simulink library "AerialManipulation"  (R2016b)
settings: Solver=VariableStepAuto  StartTime=0.0  StopTime=10.0  RelTol=1e-3
undefined symbols (not defined in the file): l
libraries: AerialManipulation x4, aerolibutil x2
settings Model: Creator=Administrator  LastModifiedBy=Administrator

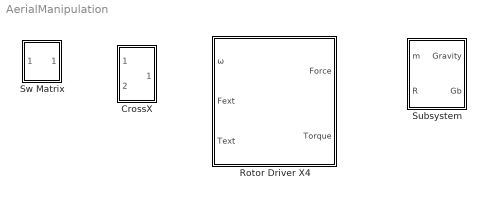
== system AerialManipulation ==
  CrossX : Subsystem
      mask help: 实现向量叉乘 V×P
      mask Display: fprintf('×\nCross');
  Rotor Driver X4 : Subsystem  mask{l=0.18, Fe=[ [0;0;1],[0;0;1],[0;0;1],[0;0;1] ], r=[ [l;0;0],[0;l;0],[-l;0;0],[0;-l;0] ], Td=[ [0;0;1], [0;0;-1],[0;0;1],[0;0;-1] ], Kct=3.16e-05, Ktf=0.01}
      mask prompts: l "length of Arm of force"; Fe "direction of vector"; r "position the force"; Td "direction of counter torque"; Kct "coefficient of counter torque"; Ktf "coefficient of thrust force"
      mask help:
      | 四旋翼的驱动模型
      | 根据四个电机的转速ω计算相应的力与力矩
      mask Display:
      | fprintf('RotorDriverX4');
      | port_label('input',1,'ω','texmode','on');
      | port_label('input',2,'Fext','texmode','on');
      | port_label('input',3,'Text','texmode','on');
      | 
      | port_label('output',1,'F','texmode','on');
      | port_label('output',2,'Torque','texmode','on');
  Subsystem : Subsystem
      mask help: 根据质量m和旋转矩阵R计算重力G和在刚体下的表示Gb
      mask Display:
      | fprintf('Gravity');
      | port_label('input',1,'m','texmode','on');
      | port_label('input',2,'R','texmode','on');
      | 
      | port_label('output',1,'G','texmode','on');
      | port_label('output',2,'Gb','texmode','on');
  Sw Matrix : Subsystem
      mask help:
      | 将一个3×1 v 的向量转为3×3矩阵Sw(v)
      | v×P=Sw(v)P
      | 参看《机器人学导论》P111 (5-25)式子
      mask Display: fprintf('Sw');

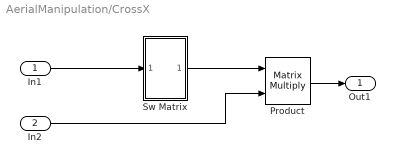
== system AerialManipulation/CrossX ==
  In1 : Inport
  In2 : Inport  Port=2
  Product : Product  Multiplication=Matrix(*)
  Sw Matrix : Subsystem
      mask help:
      | 将一个3×1 v 的向量转为3×3矩阵Sw(v)
      | v×P=Sw(v)P
      | 参看《机器人学导论》P111 (5-25)式子
      mask Display: fprintf('Sw');
  Out1 : Outport
  wires:
  In2/1 -> Product/2
  Product/1 -> Out1/1
  Sw Matrix/1(Out1) -> Product/1
  In1/1 -> Sw Matrix/1(In1)

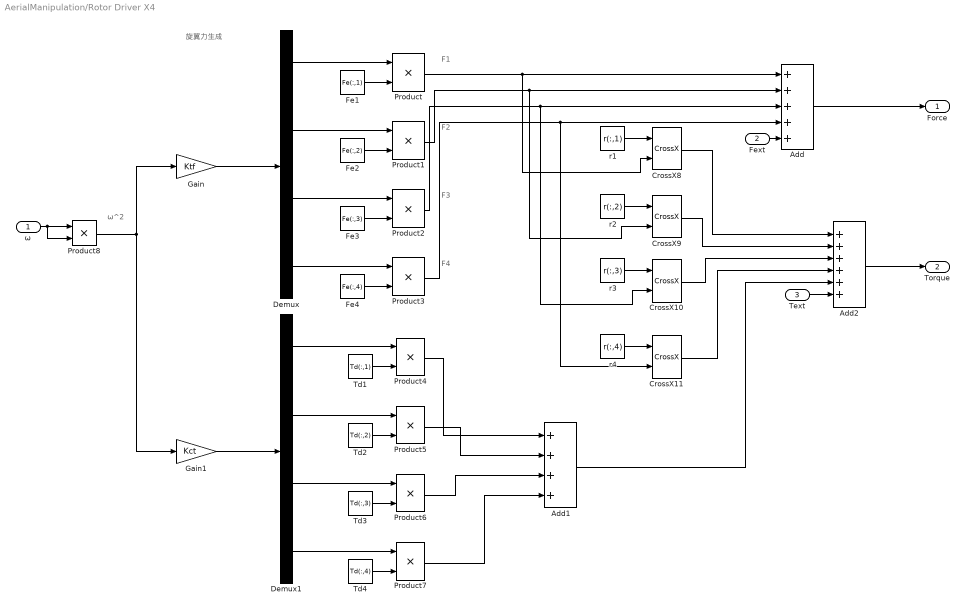
== system AerialManipulation/Rotor Driver X4 ==
  note: F4
  note: F3
  note: F2
  note: F1
  note: 旋翼力生成
  note: ω^2
  ω : Inport
  Fext : Inport  Port=2
  Text : Inport  Port=3
  Add : Sum  Inputs=+++++
  Add1 : Sum  Inputs=++++
  Add2 : Sum  Inputs=++++++
  CrossX{8..11} (4 alike) : AerialManipulation/CrossX
  Demux : Demux
  Demux1 : Demux
  Fe1 : Constant  Value=Fe(:,1)  VectorParams1D=off
  Fe2 : Constant  Value=Fe(:,2)  VectorParams1D=off
  Fe3 : Constant  Value=Fe(:,3)  VectorParams1D=off
  Fe4 : Constant  Value=Fe(:,4)
  Gain : Gain  Gain=Ktf
  Gain1 : Gain  Gain=Kct
  Product{,1..8} (9 alike) : Product
  Td1 : Constant  Value=Td(:,1)  VectorParams1D=off
  Td2 : Constant  Value=Td(:,2)  VectorParams1D=off
  Td3 : Constant  Value=Td(:,3)  VectorParams1D=off
  Td4 : Constant  Value=Td(:,4)  VectorParams1D=off
  r1 : Constant  Value=r(:,1)  VectorParams1D=off
  r2 : Constant  Value=r(:,2)  VectorParams1D=off
  r3 : Constant  Value=r(:,3)  VectorParams1D=off
  r4 : Constant  Value=r(:,4)  VectorParams1D=off
  Force : Outport
  Torque : Outport  Port=2
  wires:
  Add2/1 -> Torque/1
  Text/1 -> Add2/6
  CrossX11/1 -> Add2/4
  CrossX10/1 -> Add2/3
  CrossX9/1 -> Add2/2
  CrossX8/1 -> Add2/1
  Add1/1 -> Add2/5
  Product7/1 -> Add1/4
  Product6/1 -> Add1/3
  Product5/1 -> Add1/2
  Product4/1 -> Add1/1
  r4/1 -> CrossX11/1
  Product3/1 -> Add/4, CrossX11/2
  r3/1 -> CrossX10/1
  Product2/1 -> Add/3, CrossX10/2
  r2/1 -> CrossX9/1
  Product1/1 -> CrossX9/2, Add/2
  r1/1 -> CrossX8/1
  Td4/1 -> Product7/2
  Demux1/4 -> Product7/1
  Td3/1 -> Product6/2
  Demux1/3 -> Product6/1
  Td2/1 -> Product5/2
  Demux1/2 -> Product5/1
  Td1/1 -> Product4/2
  Demux1/1 -> Product4/1
  Gain1/1 -> Demux1/1
  Product8/1 -> Gain/1, Gain1/1
  ω/1 -> Product8/2, Product8/1
  Add/1 -> Force/1
  Fext/1 -> Add/5
  Product/1 -> CrossX8/2, Add/1
  Demux/4 -> Product3/1
  Fe2/1 -> Product1/2
  Demux/2 -> Product1/1
  Fe1/1 -> Product/2
  Demux/1 -> Product/1
  Gain/1 -> Demux/1
  Demux/3 -> Product2/1
  Fe3/1 -> Product2/2
  Fe4/1 -> Product3/2

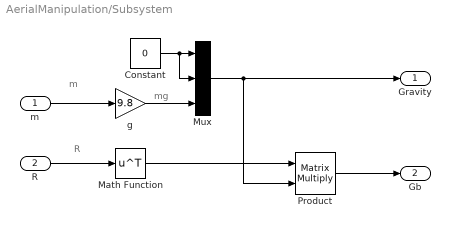
== system AerialManipulation/Subsystem ==
  note: R
  note: mg
  note: m
  m : Inport
  R : Inport  Port=2
  Constant : Constant  Value=0
  Math Function : Math  Operator=transpose  SaturateOnIntegerOverflow=on
  Mux : Mux  Inputs=3
  Product : Product  Multiplication=Matrix(*)
  g : Gain  Gain=9.8
  Gravity : Outport
  Gb : Outport  Port=2
  wires:
  Product/1 -> Gb/1
  Constant/1 -> Mux/1, Mux/2
  g/1 -> Mux/3
  m/1 -> g/1
  Math Function/1 -> Product/1
  R/1 -> Math Function/1
  Mux/1 -> Product/2, Gravity/1

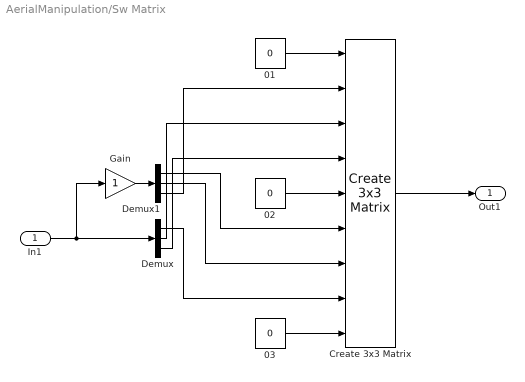
== system AerialManipulation/Sw Matrix ==
  In1 : Inport
  01 : Constant  Value=0  VectorParams1D=off
  02 : Constant  Value=0  VectorParams1D=off
  03 : Constant  Value=0  VectorParams1D=off
  Create 3x3 Matrix : aerolibutil/Create 3x3 Matrix
  Demux : Demux  Outputs=3
  Demux1 : Demux  Outputs=3
  Gain : Gain
  Out1 : Outport
  wires:
  02/1 -> Create 3x3 Matrix/5
  01/1 -> Create 3x3 Matrix/1
  Gain/1 -> Demux1/1
  Demux/3 -> Create 3x3 Matrix/4
  Demux/2 -> Create 3x3 Matrix/3
  Create 3x3 Matrix/1 -> Out1/1
  03/1 -> Create 3x3 Matrix/9
  Demux/1 -> Create 3x3 Matrix/8
  Demux1/3 -> Create 3x3 Matrix/2
  In1/1 -> Demux/1, Gain/1
  Demux1/2 -> Create 3x3 Matrix/7
  Demux1/1 -> Create 3x3 Matrix/6

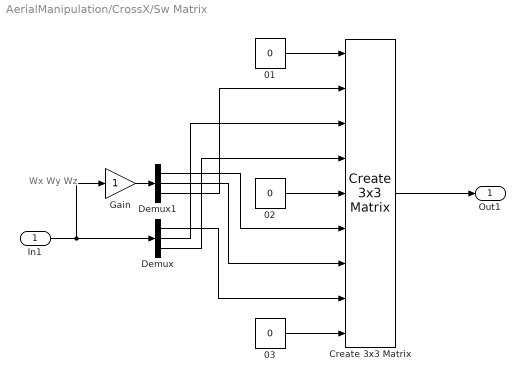
== system AerialManipulation/CrossX/Sw Matrix ==
  note: Wx
      | Wy
      | Wz
  In1 : Inport
  01 : Constant  Value=0  VectorParams1D=off
  02 : Constant  Value=0  VectorParams1D=off
  03 : Constant  Value=0  VectorParams1D=off
  Create 3x3 Matrix : aerolibutil/Create 3x3 Matrix
  Demux : Demux  Outputs=3
  Demux1 : Demux  Outputs=3
  Gain : Gain
  Out1 : Outport
  wires:
  02/1 -> Create 3x3 Matrix/5
  01/1 -> Create 3x3 Matrix/1
  Gain/1 -> Demux1/1
  Demux/3 -> Create 3x3 Matrix/4
  Demux/2 -> Create 3x3 Matrix/3
  Create 3x3 Matrix/1 -> Out1/1
  03/1 -> Create 3x3 Matrix/9
  Demux/1 -> Create 3x3 Matrix/8
  Demux1/3 -> Create 3x3 Matrix/2
  In1/1 -> Demux/1, Gain/1
  Demux1/2 -> Create 3x3 Matrix/7
  Demux1/1 -> Create 3x3 Matrix/6
